simulink model "BenchmarkModel_Dynamic_TestCase"  (R2020a)
settings: Solver=ode45  StartTime=0.0  StopTime=5  RelTol=1e-3
undefined symbols (not defined in the file): Angle, D1, Delta, find_system, Magnitude
libraries: powerlib x91, powerlib_meascontrol x31, simulink x6, dspsrcs4 x3, dspsigops x2, sps_avr x1
(part 2 of 3)

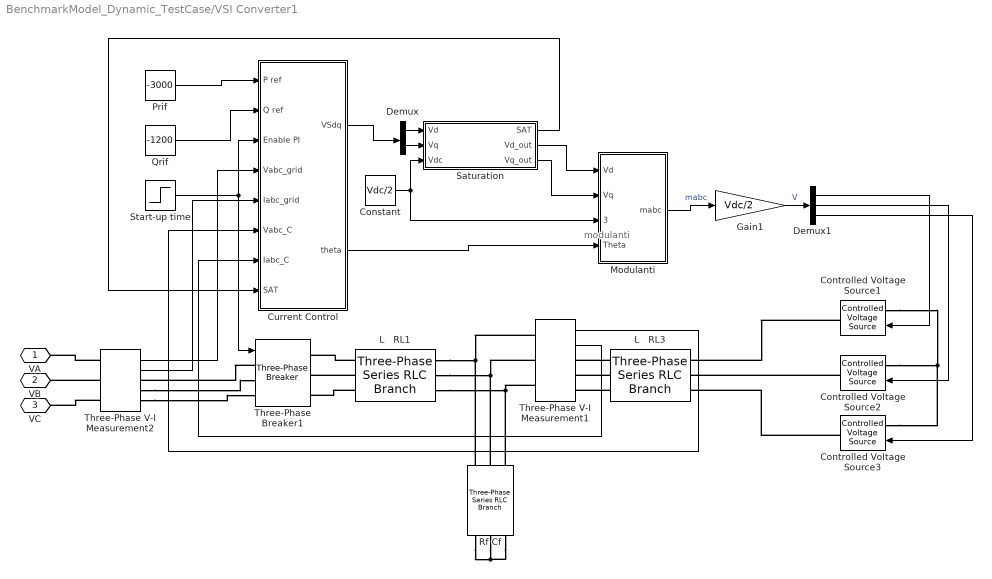
== system BenchmarkModel_Dynamic_TestCase/VSI Converter1 ==
  note: modulanti
  Constant : Constant  Value=Vdc/2
  Controlled Voltage Source1 : powerlib/Electrical Sources/Controlled Voltage Source  Initialize=on  Source_Type=DC  Amplitude=0  Phase=0  Frequency=0  Measurements=None
  Controlled Voltage Source2 : powerlib/Electrical Sources/Controlled Voltage Source  Initialize=on  Source_Type=DC  Amplitude=0  Phase=0  Frequency=0  Measurements=None
  Controlled Voltage Source3 : powerlib/Electrical Sources/Controlled Voltage Source  Initialize=on  Source_Type=DC  Amplitude=0  Phase=0  Frequency=0  Measurements=None
  Current Control : Subsystem
  Demux : Demux  Outputs=2
  Demux1 : Demux  Outputs=3
  Gain1 : Gain  Gain=Vdc/2
  L	  RL1 : powerlib/Elements/Three-Phase Series RLC Branch  LConnTagsString=A|B|C  RConnTagsString=A|B|C  BranchType=L  Resistance=0  Inductance=Lf  Capacitance=100e-6  Measurements=Branch voltages
  L	  RL3 : powerlib/Elements/Three-Phase Series RLC Branch  LConnTagsString=A|B|C  RConnTagsString=A|B|C  BranchType=RL  Resistance=10e-3  Inductance=L1t  Capacitance=100e-6  Measurements=None
  Modulanti : Subsystem
  Prif : Constant  Value=-3000
  Qrif : Constant  Value=-1200
  "Rf Cf  " : powerlib/Elements/Three-Phase Series RLC Branch  LConnTagsString=A|B|C  RConnTagsString=A|B|C  BranchType=RC  Resistance=1e-3  Inductance=1e-3  Capacitance=Cf  Measurements=Branch voltages
  Saturation : MATLAB Function  TreatAsAtomicUnit=on
  Start-up time : Step  Time=0.05  SampleTime=0
  Three-Phase V-I Measurement1 : powerlib/Measurements/Three-Phase V-I Measurement  VoltageMeasurement=phase-to-phase  SetLabelV=off  LabelV=Vabc  Vpu=off  VpuLL=off  CurrentMeasurement=yes  SetLabelI=off  LabelI=Iabc  Ipu=off  Pbase=100e6  Vbase=500e3  OutputType=Complex  PhasorSimulation=off  PSBequivalent=0
  Three-Phase V-I Measurement2 : powerlib/Measurements/Three-Phase V-I Measurement  VoltageMeasurement=phase-to-phase  SetLabelV=off  LabelV=Vabc  Vpu=off  VpuLL=off  CurrentMeasurement=yes  SetLabelI=off  LabelI=Iabc  Ipu=off  Pbase=100e6  Vbase=500e3  OutputType=Complex  PhasorSimulation=off  PSBequivalent=0
  Three-Phase Breaker1 : powerlib/Elements/Three-Phase Breaker  InitialState=open  SwitchA=on  SwitchB=on  SwitchC=on  SwitchTimes="[1/60  5/60]"  External=on  BreakerResistance=0.001  SnubberResistance=1e6  SnubberCapacitance=inf  Measurements=None
  VA : PMIOPort  Side=Left
  VB : PMIOPort  Port=2  Side=Left
  VC : PMIOPort  Port=3  Side=Left
  wires:
  Constant/1 -> Modulanti/3(Vdcbus), Saturation/3(Vdc)
  Saturation/1(SAT) -> Current Control/8(SAT)
  Start-up time/1 -> Three-Phase Breaker1/1, Current Control/3(Enable PI)
  Current Control/1(VSdq) -> Demux/1
  Demux/1 -> Saturation/1(Vd)
  Demux/2 -> Saturation/2(Vq)
  Saturation/2(Vd_out) -> Modulanti/1(Vd)
  Saturation/3(Vq_out) -> Modulanti/2(Vq)
  Modulanti/1(mabc) -> Gain1/1  "mabc"
  Demux1/1 -> Controlled Voltage Source1/1
  Demux1/2 -> Controlled Voltage Source2/1
  Demux1/3 -> Controlled Voltage Source3/1
  Gain1/1 -> Demux1/1  "V"
  Prif/1 -> Current Control/1(P ref)
  Qrif/1 -> Current Control/2(Q ref)
  Three-Phase V-I Measurement2/2 -> Current Control/5(Iabc_grid)
  Three-Phase V-I Measurement2/1 -> Current Control/4(Vabc_grid)
  Three-Phase V-I Measurement1/2 -> Current Control/7(Iabc_C)
  Three-Phase V-I Measurement1/1 -> Current Control/6(Vabc_C)
  Current Control/2(theta) -> Modulanti/4(Theta)
  connections:
  L	  RL1/LConn3 -- Three-Phase V-I Measurement1/LConn3 -- "Rf Cf  "/LConn3
  "Rf Cf  "/RConn1 -- "Rf Cf  "/RConn3 -- "Rf Cf  "/RConn2
  L	  RL1/LConn1 -- Three-Phase V-I Measurement1/LConn1 -- "Rf Cf  "/LConn1
  L	  RL1/LConn2 -- Three-Phase V-I Measurement1/LConn2 -- "Rf Cf  "/LConn2
  Controlled Voltage Source3/RConn1 -- L	  RL3/LConn3
  Controlled Voltage Source1/RConn1 -- L	  RL3/LConn1
  L	  RL1/RConn1 -- Three-Phase Breaker1/RConn1
  L	  RL1/RConn2 -- Three-Phase Breaker1/RConn2
  L	  RL1/RConn3 -- Three-Phase Breaker1/RConn3
  Three-Phase V-I Measurement2/LConn3 -- VC/RConn1
  Three-Phase V-I Measurement2/LConn2 -- VB/RConn1
  Three-Phase V-I Measurement2/LConn1 -- VA/RConn1
  Controlled Voltage Source2/LConn1 -- Controlled Voltage Source1/LConn1 -- Controlled Voltage Source3/LConn1
  Controlled Voltage Source2/RConn1 -- L	  RL3/LConn2
  Three-Phase Breaker1/LConn1 -- Three-Phase V-I Measurement2/RConn1
  L	  RL3/RConn1 -- Three-Phase V-I Measurement1/RConn1
  L	  RL3/RConn2 -- Three-Phase V-I Measurement1/RConn2
  L	  RL3/RConn3 -- Three-Phase V-I Measurement1/RConn3
  Three-Phase V-I Measurement2/RConn2 -- Three-Phase Breaker1/LConn2
  Three-Phase V-I Measurement2/RConn3 -- Three-Phase Breaker1/LConn3

== system BenchmarkModel_Dynamic_TestCase/Zero-crossing detector ==
  Ground2 : powerlib/Elements/Ground  LConnTagsString=a
  To Workspace5 : ToWorkspace  VariableName=Crossing_Inv  SaveFormat=Timeseries  SampleTime=-1
  Voltage Measurement2 : powerlib/Measurements/Voltage Measurement  PhasorSimulation=off  OutputType=Complex  PSBequivalent=0
  Zero Crossing1 : dspsigops/Zero Crossing  InputProcessing=Columns as channels (frame based)
      settings: SourceProductBaseCode=DS
  v : PMIOPort  Side=Left
  wires:
  Voltage Measurement2/1 -> Zero Crossing1/1
  Zero Crossing1/1 -> To Workspace5/1
  connections:
  Ground2/LConn1 -- Voltage Measurement2/LConn2
  v/RConn1 -- Voltage Measurement2/LConn1

== system BenchmarkModel_Dynamic_TestCase/ZeroCrossing Detector ==
  Ground1 : powerlib/Elements/Ground  LConnTagsString=a
  To Workspace4 : ToWorkspace  VariableName=Crossing  SaveFormat=Timeseries  SampleTime=-1
  Voltage Measurement1 : powerlib/Measurements/Voltage Measurement  PhasorSimulation=off  OutputType=Complex  PSBequivalent=0
  Zero Crossing : dspsigops/Zero Crossing  InputProcessing=Columns as channels (frame based)
      settings: SourceProductBaseCode=DS
  fr : PMIOPort  Side=Left
  wires:
  Zero Crossing/1 -> To Workspace4/1
  Voltage Measurement1/1 -> Zero Crossing/1
  connections:
  Ground1/LConn1 -- Voltage Measurement1/LConn2
  fr/RConn1 -- Voltage Measurement1/LConn1

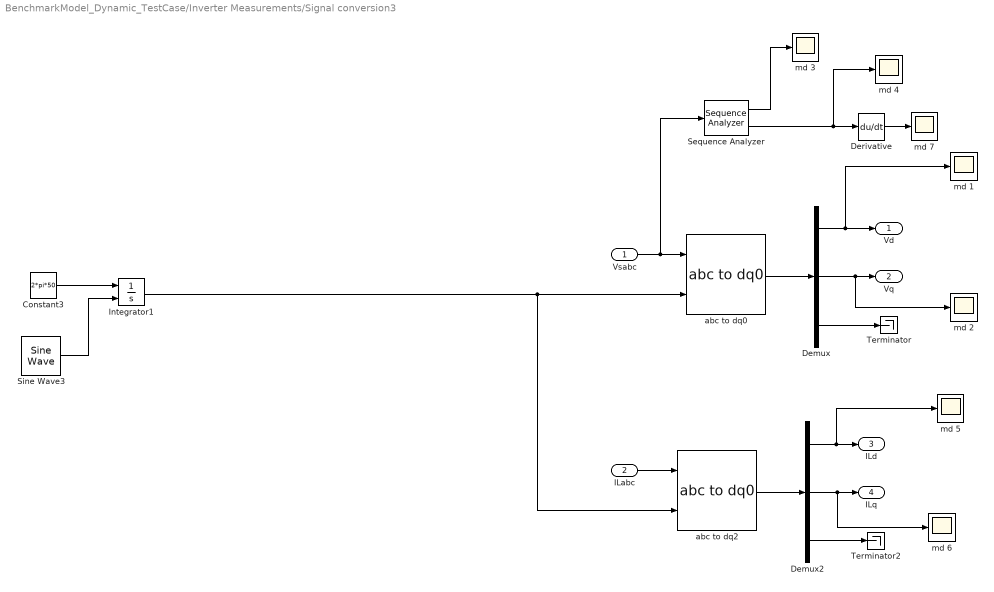
== system BenchmarkModel_Dynamic_TestCase/Inverter Measurements/Signal conversion3 ==
  Vsabc : Inport
  ILabc : Inport  Port=2
  Constant3 : Constant  Value=2*pi*50
  Demux : Demux  Outputs=3
  Demux2 : Demux  Outputs=3
  Derivative : Derivative
  Integrator1 : Integrator  ExternalReset=rising
  Sequence Analyzer : powerlib_meascontrol/Measurements/Sequence Analyzer  Freq=50  n=1  seq=Positive Negative Zero  InInit=[1, 0]  Ts=0
      settings: SourceProductBaseCode=PS
  Sine Wave3 : dspsrcs4/Sine Wave  Amplitude=1  Frequency=50  Phase=0  SampleMode=Continuous  OutComplex=Real  CompMethod=Trigonometric fcn  TableSize=Speed  SampleTime=5e-6  SamplesPerFrame=1  ResetState=Restart at time zero  OutputFrames=on  dataType=double  wordLen=16  udDataType=sfix(16)  fracBitsMode=Best precision  numFracBits=15  OutDataTypeStr=double  LastOutDataTypeStr=double
  Terminator : Terminator
  Terminator2 : Terminator
  abc to dq0 : powerlib_meascontrol/Transformations/abc to dq0  Alignment=90 degrees behind phase A axis
  abc to dq2 : powerlib_meascontrol/Transformations/abc to dq0  Alignment=90 degrees behind phase A axis
  md {1..7} (7 alike) : Scope
  Vd : Outport
  Vq : Outport  Port=2
  ILd : Outport  Port=3
  ILq : Outport  Port=4
  wires:
  Vsabc/1 -> Sequence Analyzer/1, abc to dq0/1
  Demux2/1 -> ILd/1, md 5/1
  Integrator1/1 -> abc to dq2/2, abc to dq0/2
  ILabc/1 -> abc to dq2/1
  Demux2/3 -> Terminator2/1
  Demux/3 -> Terminator/1
  Constant3/1 -> Integrator1/1
  abc to dq0/1 -> Demux/1
  abc to dq2/1 -> Demux2/1
  Demux/1 -> Vd/1, md 1/1
  Demux/2 -> Vq/1, md 2/1
  Demux2/2 -> ILq/1, md 6/1
  Sine Wave3/1 -> Integrator1/2
  Sequence Analyzer/1 -> md 3/1
  Sequence Analyzer/2 -> Derivative/1, md 4/1
  Derivative/1 -> md 7/1

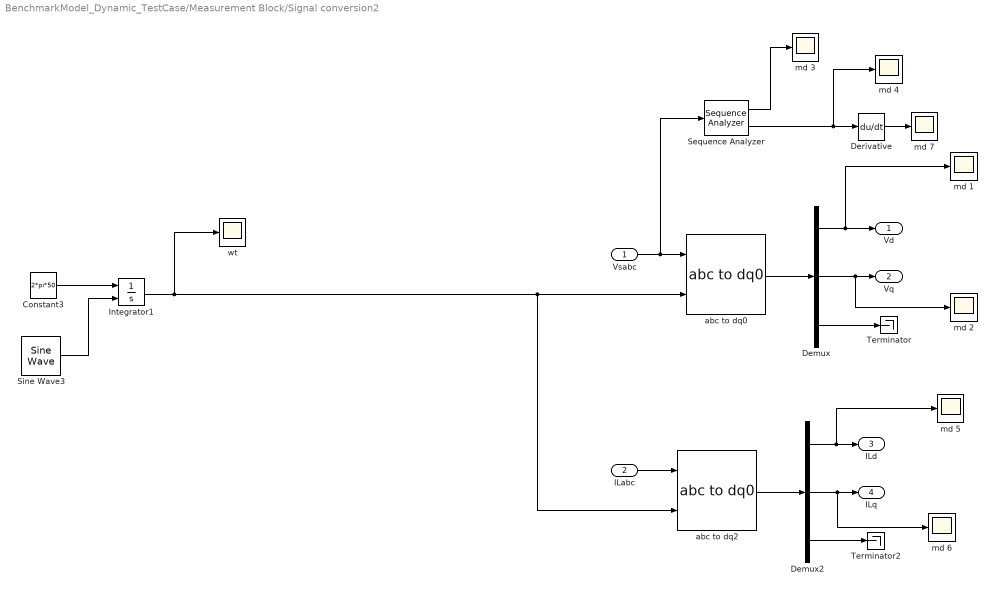
== system BenchmarkModel_Dynamic_TestCase/Measurement Block/Signal conversion2 ==
  Vsabc : Inport
  ILabc : Inport  Port=2
  Constant3 : Constant  Value=2*pi*50
  Demux : Demux  Outputs=3
  Demux2 : Demux  Outputs=3
  Derivative : Derivative
  Integrator1 : Integrator  ExternalReset=rising
  Sequence Analyzer : powerlib_meascontrol/Measurements/Sequence Analyzer  Freq=50  n=1  seq=Positive Negative Zero  InInit=[1, 0]  Ts=0
      settings: SourceProductBaseCode=PS
  Sine Wave3 : dspsrcs4/Sine Wave  Amplitude=1  Frequency=50  Phase=0  SampleMode=Continuous  OutComplex=Real  CompMethod=Trigonometric fcn  TableSize=Speed  SampleTime=5e-6  SamplesPerFrame=1  ResetState=Restart at time zero  OutputFrames=on  dataType=double  wordLen=16  udDataType=sfix(16)  fracBitsMode=Best precision  numFracBits=15  OutDataTypeStr=double  LastOutDataTypeStr=double
  Terminator : Terminator
  Terminator2 : Terminator
  abc to dq0 : powerlib_meascontrol/Transformations/abc to dq0  Alignment=90 degrees behind phase A axis
  abc to dq2 : powerlib_meascontrol/Transformations/abc to dq0  Alignment=90 degrees behind phase A axis
  md {1..7} (7 alike) : Scope
  wt : Scope
  Vd : Outport
  Vq : Outport  Port=2
  ILd : Outport  Port=3
  ILq : Outport  Port=4
  wires:
  Vsabc/1 -> Sequence Analyzer/1, abc to dq0/1
  Demux2/1 -> ILd/1, md 5/1
  Integrator1/1 -> abc to dq2/2, abc to dq0/2, wt/1
  ILabc/1 -> abc to dq2/1
  Demux2/3 -> Terminator2/1
  Demux/3 -> Terminator/1
  Constant3/1 -> Integrator1/1
  abc to dq0/1 -> Demux/1
  abc to dq2/1 -> Demux2/1
  Demux/1 -> Vd/1, md 1/1
  Demux/2 -> Vq/1, md 2/1
  Demux2/2 -> ILq/1, md 6/1
  Sine Wave3/1 -> Integrator1/2
  Sequence Analyzer/1 -> md 3/1
  Sequence Analyzer/2 -> Derivative/1, md 4/1
  Derivative/1 -> md 7/1

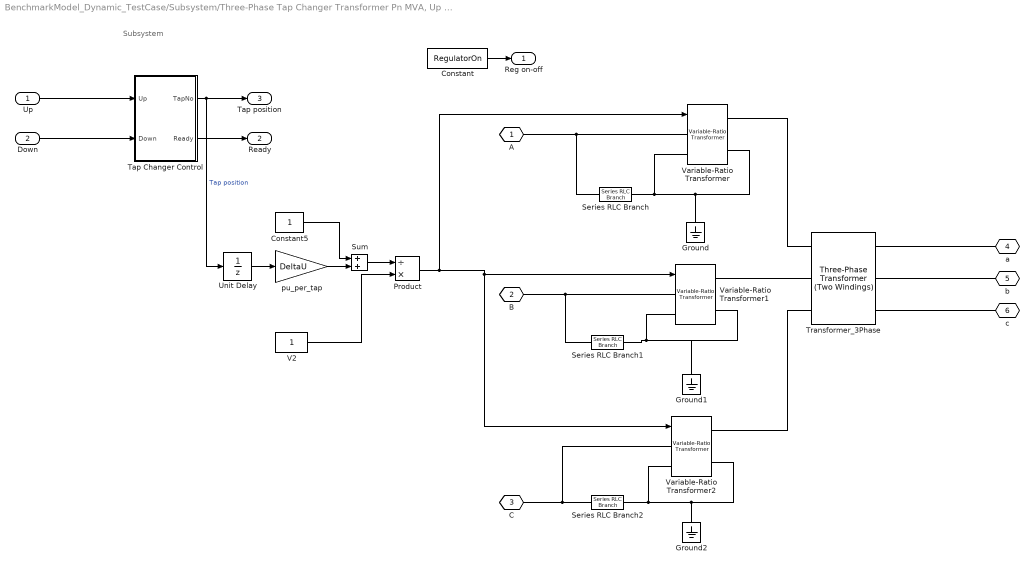
== system BenchmarkModel_Dynamic_TestCase/Subsystem/Three-Phase Tap Changer Transformer Pn MVA, Up // Us kV ==
  note: Subsystem
  Up : Inport
  Down : Inport  Port=2
  Constant : Constant  Value=RegulatorOn
  Constant5 : Constant
  Ground : powerlib/Elements/Ground  LConnTagsString=a
  Ground1 : powerlib/Elements/Ground  LConnTagsString=a
  Ground2 : powerlib/Elements/Ground  LConnTagsString=a
  Product : Product  Inputs=/*
  Series RLC Branch : powerlib/Elements/Series RLC Branch  LConnTagsString=__new0  RConnTagsString=__new0  BranchType=R  Resistance=1e7  Inductance=1e-3  SetiL0=off  InitialCurrent=0  Capacitance=1e-6  Setx0=off  InitialVoltage=0  Measurements=None
  Series RLC Branch1 : powerlib/Elements/Series RLC Branch  LConnTagsString=__new0  RConnTagsString=__new0  BranchType=R  Resistance=1e7  Inductance=1e-3  SetiL0=off  InitialCurrent=0  Capacitance=1e-6  Setx0=off  InitialVoltage=0  Measurements=None
  Series RLC Branch2 : powerlib/Elements/Series RLC Branch  LConnTagsString=__new0  RConnTagsString=__new0  BranchType=R  Resistance=1e7  Inductance=1e-3  SetiL0=off  InitialCurrent=0  Capacitance=1e-6  Setx0=off  InitialVoltage=0  Measurements=None
  Sum : Sum
  Tap Changer Control : Subsystem  mask(Tap Changer Control){MinMaxTap=TapMinMax, InitialPosition=InitialTap, MecDelay=TapSelectionTime}
      mask prompts: MinMaxTap "Minimum and maximum tap number [ Min  Max ] :"; InitialPosition "Initial tap position"; MecDelay "Mechanical delay time"
      mask init:
      | if MecDelay<=0,
      | 	MecDelay=1/60;
      | end
  Transformer_3Phase : powerlib/Elements/Three-Phase Transformer (Two Windings)  Winding1Connection=Yg  Winding2Connection=Delta (D1)  CoreType=Three single-phase transformers  SetSaturation=off  Hysteresis=off  DataFile='hysteresis'  SetInitialFlux=off  Measurements=Fluxes and magnetization currents ( Imag )  UNITS=pu  NominalPower=NominalParameters  Winding1=Winding1  Winding2=Winding2  Rm=Rmpu  Lm=Lmpu  L0=0.5  Saturation=[ 0,0 ; 0.0024,1.2 ; 1.0,1.52 ]  InitialFluxes=[ 0.8 , -0.8 , 0.7 ]  BreakLoop=off  DiscreteSolver=Trapezoidal iterative  DataType=off  TransfoNumber=1
  Unit Delay : UnitDelay  InitialCondition=InitialTap  SampleTime=50e-6  HasFrameUpgradeWarning=on
  V2 : Constant
  Variable-Ratio Transformer : powerlib/Elements/Variable-Ratio Transformer
      settings: SourceProductBaseCode=PS
  Variable-Ratio Transformer1 : powerlib/Elements/Variable-Ratio Transformer
      settings: SourceProductBaseCode=PS
  Variable-Ratio Transformer2 : powerlib/Elements/Variable-Ratio Transformer
      settings: SourceProductBaseCode=PS
  pu_per_tap : Gain  Gain=DeltaU
  A : PMIOPort  Tag=PMCPort  Side=Left
  B : PMIOPort  Tag=PMCPort  Port=2  Side=Left
  C : PMIOPort  Tag=PMCPort  Port=3  Side=Left
  a : PMIOPort  Tag=PMCPort  Port=4  Side=Right
  b : PMIOPort  Tag=PMCPort  Port=5  Side=Right
  c : PMIOPort  Tag=PMCPort  Port=6  Side=Right
  Reg on-off : Outport
  Ready : Outport  Port=2
  Tap position : Outport  Port=3
  wires:
  Constant/1 -> Reg on-off/1
  Tap Changer Control/2(Ready) -> Ready/1
  Constant5/1 -> Sum/1
  Up/1 -> Tap Changer Control/1("Up ")
  Tap Changer Control/1(TapNo) -> Unit Delay/1, Tap position/1  "Tap position"
  Unit Delay/1 -> pu_per_tap/1
  Down/1 -> Tap Changer Control/2("Down ")
  Sum/1 -> Product/1
  V2/1 -> Product/2
  pu_per_tap/1 -> Sum/2
  Product/1 -> Variable-Ratio Transformer2/1, Variable-Ratio Transformer1/1, Variable-Ratio Transformer/1
  connections:
  Transformer_3Phase/RConn1 -- a/RConn1
  Transformer_3Phase/RConn2 -- b/RConn1
  Transformer_3Phase/RConn3 -- c/RConn1
  Transformer_3Phase/LConn2 -- Variable-Ratio Transformer1/RConn1
  Transformer_3Phase/LConn3 -- Variable-Ratio Transformer2/RConn1
  Transformer_3Phase/LConn1 -- Variable-Ratio Transformer/RConn1
  Series RLC Branch1/LConn1 -- B/RConn1 -- Variable-Ratio Transformer1/LConn1
  Variable-Ratio Transformer/LConn1 -- A/RConn1 -- Series RLC Branch/LConn1
  Series RLC Branch2/LConn1 -- Variable-Ratio Transformer2/LConn1 -- C/RConn1
  Ground2/LConn1 -- Variable-Ratio Transformer2/LConn2 -- Series RLC Branch2/RConn1 -- Variable-Ratio Transformer2/RConn2
  Series RLC Branch1/RConn1 -- Variable-Ratio Transformer1/RConn2 -- Ground1/LConn1 -- Variable-Ratio Transformer1/LConn2
  Ground/LConn1 -- Variable-Ratio Transformer/LConn2 -- Series RLC Branch/RConn1 -- Variable-Ratio Transformer/RConn2

== system BenchmarkModel_Dynamic_TestCase/Subsystem/Voltage regulator ==
  Vmes (pu) : Inport
  Ready : Inport  Port=2
  RegOn : Inport  Port=3
  Dead Zone : DeadZone  LowerValue=-DeadBand/2  UpperValue=+DeadBand/2  SaturateOnIntegerOverflow=on
  Discrete Variable Time Delay1 : powerlib_meascontrol/Additional Components/Discrete Variable Time Delay  MaxDelay=3/60+50e-6  InitialValue=1  Ts=50e-6  DFT=on
      settings: SourceProductBaseCode=PS
  Logical Operator : Logic  AllPortsSameDT=off
  Logical Operator1 : Logic  AllPortsSameDT=off
  On Delay : powerlib_meascontrol/Logic/On Delay  DelayType=On delay  delay=TimeDelay  ic=0  Ts=50e-6
  On Delay1 : powerlib_meascontrol/Logic/On Delay  DelayType=On delay  delay=TimeDelay  ic=0  Ts=50e-6
  Relational Operator : RelationalOperator  Operator=<  RndMeth=Nearest
  Relational Operator1 : RelationalOperator  Operator=>  RndMeth=Nearest
  Scope : Scope  Commented=on  NumInputPorts=2
  Sum : Sum  Inputs=|+-  SaturateOnIntegerOverflow=on
  Switch : Switch  Threshold=1.5  SaturateOnIntegerOverflow=on
  Vref : Constant  Value=Vref
  Vref1 : Constant  Value=0
  Vref2 : Constant  Value=0
  Vref3 : Constant  Value=0
  Vref4 : Constant  Value=3/60
  Up : Outport  VectorParamsAs1DForOutWhenUnconnected=off
  Down : Outport  Port=2  VectorParamsAs1DForOutWhenUnconnected=off
  wires:
  Vref4/1 -> Discrete Variable Time Delay1/2
  Discrete Variable Time Delay1/1 -> Logical Operator/2, Logical Operator1/1
  Vref3/1 -> Relational Operator1/2
  On Delay1/1 -> Down/1
  Logical Operator1/1 -> On Delay1/1
  Relational Operator1/1 -> Logical Operator1/2
  On Delay/1 -> Up/1
  Logical Operator/1 -> On Delay/1
  Ready/1 -> Discrete Variable Time Delay1/1
  Relational Operator/1 -> Logical Operator/1
  Vref1/1 -> Relational Operator/2
  Dead Zone/1 -> Scope/2, Relational Operator/1, Relational Operator1/1
  Vmes (pu)/1 -> Sum/2
  Vref/1 -> Sum/1
  Sum/1 -> Switch/1
  Switch/1 -> Scope/1, Dead Zone/1  "bfor"
  RegOn/1 -> Switch/2
  Vref2/1 -> Switch/3

== system BenchmarkModel_Dynamic_TestCase/Subsystem1/POWER CONVERTER1 ==
  phase3 : Inport
  Add : Sum
  Add2 : Sum
  Add4 : Sum
  Ampl : Constant  Value=20000*sqrt(2)/sqrt(3)
  Product : Product
  Product1 : Product
  Product2 : Product
  Sin : Trigonometry
  Sin1 : Trigonometry
  Sin2 : Trigonometry
  phase : Constant  Value=0
  phase1 : Constant  Value=-120*pi/180
  phase2 : Constant  Value=-240*pi/180
  Phase A : Outport
  Phase B : Outport  Port=2
  Phase C : Outport  Port=3
  wires:
  phase/1 -> Add/1
  Add/1 -> Sin/1
  phase1/1 -> Add2/1
  Add2/1 -> Sin1/1
  phase2/1 -> Add4/1
  Add4/1 -> Sin2/1
  phase3/1 -> Add/2, Add4/2, Add2/2
  Ampl/1 -> Product2/1, Product1/1, Product/1
  Product1/1 -> Phase B/1
  Product2/1 -> Phase C/1
  Product/1 -> Phase A/1
  Sin/1 -> Product/2
  Sin1/1 -> Product1/2
  Sin2/1 -> Product2/2

== system BenchmarkModel_Dynamic_TestCase/Subsystem1/Phase calculator1 ==
  f1 : Inport
  Add3 : Sum  Inputs=+-
  Gain : Gain  Gain=2*pi
  Integrator : Integrator
  f : Constant  Value=0
  phase : Outport
  wires:
  Add3/1 -> Gain/1
  f/1 -> Add3/2
  f1/1 -> Add3/1
  Integrator/1 -> phase/1
  Gain/1 -> Integrator/1

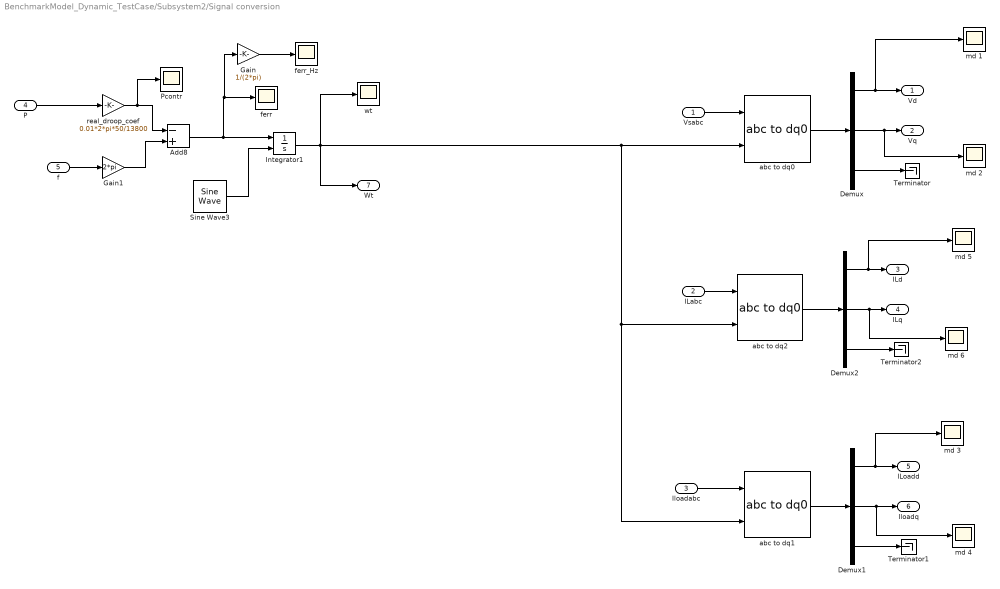
== system BenchmarkModel_Dynamic_TestCase/Subsystem2/Signal conversion ==
  Vsabc : Inport
  ILabc : Inport  Port=2
  Iloadabc : Inport  Port=3
  P : Inport  Port=4
  f : Inport  Port=5
  Add8 : Sum  Inputs=-+
  Demux : Demux  Outputs=3
  Demux1 : Demux  Outputs=3
  Demux2 : Demux  Outputs=3
  Gain : Gain  Gain=1/(2*pi)
  Gain1 : Gain  Gain=2*pi
  Integrator1 : Integrator  ExternalReset=rising
  Pcontr : Scope
  Sine Wave3 : dspsrcs4/Sine Wave  Amplitude=1  Frequency=50  Phase=0  SampleMode=Continuous  OutComplex=Real  CompMethod=Trigonometric fcn  TableSize=Speed  SampleTime=5e-6  SamplesPerFrame=1  ResetState=Restart at time zero  OutputFrames=on  dataType=double  wordLen=16  udDataType=sfix(16)  fracBitsMode=Best precision  numFracBits=15  OutDataTypeStr=double  LastOutDataTypeStr=double
  Terminator : Terminator
  Terminator1 : Terminator
  Terminator2 : Terminator
  abc to dq0 : powerlib_meascontrol/Transformations/abc to dq0  Alignment=90 degrees behind phase A axis
  abc to dq1 : powerlib_meascontrol/Transformations/abc to dq0  Alignment=90 degrees behind phase A axis
  abc to dq2 : powerlib_meascontrol/Transformations/abc to dq0  Alignment=90 degrees behind phase A axis
  ferr : Scope
  ferr_Hz : Scope
  md {1..6} (6 alike) : Scope
  real_droop_coef : Gain  Gain=0.01*2*pi*50/13800
  wt : Scope
  Vd : Outport
  Vq : Outport  Port=2
  ILd : Outport  Port=3
  ILq : Outport  Port=4
  ILoadd : Outport  Port=5
  Iloadq : Outport  Port=6
  Wt : Outport  Port=7
  wires:
  Vsabc/1 -> abc to dq0/1
  Demux2/1 -> ILd/1, md 5/1
  Integrator1/1 -> Wt/1, abc to dq1/2, abc to dq2/2, abc to dq0/2, wt/1
  Demux1/3 -> Terminator1/1
  Demux1/1 -> ILoadd/1, md 3/1
  Iloadabc/1 -> abc to dq1/1
  ILabc/1 -> abc to dq2/1
  Demux1/2 -> Iloadq/1, md 4/1
  Demux2/3 -> Terminator2/1
  Demux/3 -> Terminator/1
  abc to dq1/1 -> Demux1/1
  abc to dq0/1 -> Demux/1
  abc to dq2/1 -> Demux2/1
  Demux/1 -> Vd/1, md 1/1
  Demux/2 -> Vq/1, md 2/1
  Demux2/2 -> ILq/1, md 6/1
  Sine Wave3/1 -> Integrator1/2
  P/1 -> real_droop_coef/1
  Gain1/1 -> Add8/2
  real_droop_coef/1 -> Pcontr/1, Add8/1
  Add8/1 -> Gain/1, ferr/1, Integrator1/1
  Gain/1 -> ferr_Hz/1
  f/1 -> Gain1/1

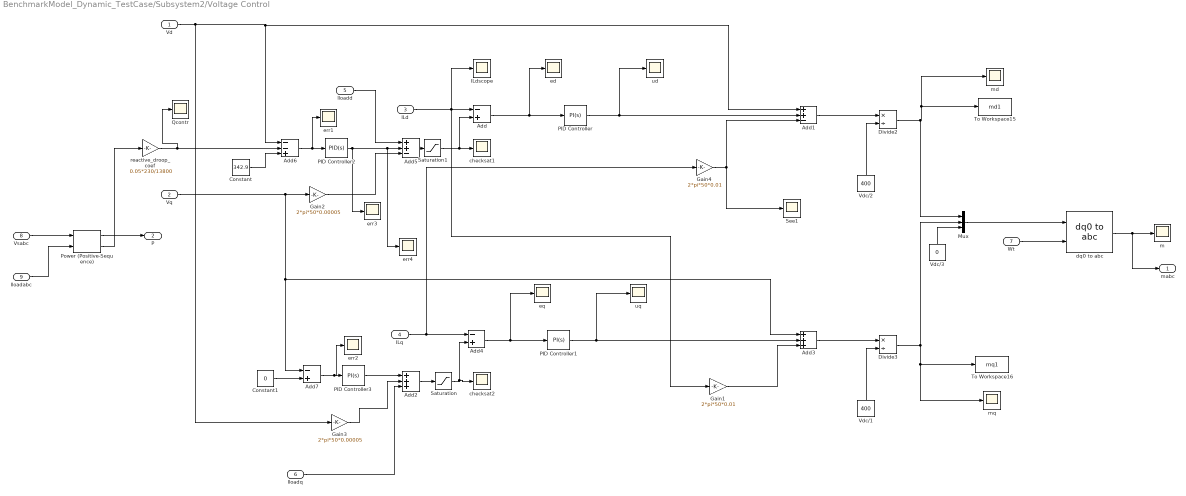
== system BenchmarkModel_Dynamic_TestCase/Subsystem2/Voltage Control ==
  Vd : Inport
  Vq : Inport  Port=2
  ILd : Inport  Port=3
  ILq : Inport  Port=4
  Iloadd : Inport  Port=5
  Iloadq : Inport  Port=6
  Wt : Inport  Port=7
  Vsabc : Inport  Port=8
  Iloadabc : Inport  Port=9
  Add : Sum  Inputs=-+
  Add1 : Sum  Inputs=++-
  Add2 : Sum  Inputs=+++
  Add3 : Sum  Inputs=+++
  Add4 : Sum  Inputs=-+
  Add5 : Sum  Inputs=++-
  Add6 : Sum  Inputs=--+
  Add7 : Sum  Inputs=-+
  Constant : Constant  Value=342.9
  Constant1 : Constant  Value=0
  Divide2 : Product  Inputs=*/
  Divide3 : Product  Inputs=*/
  Gain1 : Gain  Gain=2*pi*50*0.01
  Gain2 : Gain  Gain=2*pi*50*0.00005
  Gain3 : Gain  Gain=2*pi*50*0.00005
  Gain4 : Gain  Gain=2*pi*50*0.01
  ILdscope : Scope
  Mux : Mux  Inputs=3
  PID Controller : simulink/Continuous/PID Controller  Controller=PI  Form=Parallel  TimeDomain=Continuous-time  UseExternalTs=off  SampleTime=-1  IntegratorMethod=Forward Euler  FilterMethod=Forward Euler  ControllerParametersSource=internal  P=20  I=100  D=0  UseFilter=on  N=100  TunerSelectOption=Transfer Function Based (PID Tuner App)  InitialConditionSource=internal  InitialConditionForIntegrator=0  InitialConditionForFilter=0  DifferentiatorICPrevScaledInput=0  ExternalReset=none  TrackingMode=off  Kt=1  LimitOutput=off  UpperSaturationLimit=inf  LowerSaturationLimit=-inf  LinearizeAsGain=on  AntiWindupMode=none  Kb=1  POutMin=[]  POutMax=[]  IOutMin=[]  IOutMax=[]  DOutMin=[]  DOutMax=[]  NOutMin=[]  NOutMax=[]  SumOutMin=[]  SumOutMax=[]  SaturationOutMin=[]  SaturationOutMax=[]  PParamMin=[]  PParamMax=[]  IParamMin=[]  IParamMax=[]  DParamMin=[]  DParamMax=[]  NParamMin=[]  NParamMax=[]  KbParamMin=[]  KbParamMax=[]  KtParamMin=[]  KtParamMax=[]  KbOutMin=[]  KbOutMax=[]  KtOutMin=[]  KtOutMax=[]  IntegratorOutMin=[]  IntegratorOutMax=[]  FilterOutMin=[]  FilterOutMax=[]  SumI1OutMin=[]  SumI1OutMax=[]  SumI2OutMin=[]  SumI2OutMax=[]  SumI3OutMin=[]  SumI3OutMax=[]  SumI4OutMin=[]  SumI4OutMax=[]  SumDOutMin=[]  SumDOutMax=[]  DifferentiatorOutMin=[]  DifferentiatorOutMax=[]  FilterDiffOutCoefMin=[]  FilterDiffOutCoefMax=[]  ReciprocalOutMin=[]  ReciprocalOutMax=[]  SumDenOutMin=[]  SumDenOutMax=[]  SumNumOutMin=[]  SumNumOutMax=[]  DivideOutMin=[]  DivideOutMax=[]  UdiffTsProdOutMin=[]  UdiffTsProdOutMax=[]  NTsProdOutMin=[]  NTsProdOutMax=[]  UintegralTsProdOutMin=[]  UintegralTsProdOutMax=[]  UngainTsProdOutMin=[]  UngainTsProdOutMax=[]  IntegratorContinuousStateAttributes=''  IntegratorStateMustResolveToSignalObject=off  IntegratorRTWStateStorageClass=Auto  FilterContinuousStateAttributes=''  FilterStateMustResolveToSignalObject=off  FilterRTWStateStorageClass=Auto  ParallelPVariant=InternalParameters  IdealPVariant=Disabled  IVariant=InternalParameters  DVariant=Disabled  IntegratorVariant=Continuous  SatVariant=Disabled  AWVariant=Passthrough  PCopyVariant=Disabled  TRVariant=Disabled  FdbkBlocksVariant=Forward  IdealPFdbkVariant=Disabled  SatFdbkVariant=Disabled  DerivativeFilterVariant=Disabled  NVariant=Disabled  NCopyVariant=Disabled_SignalSpec  FilterICVariant=Disabled  IntegratorICVariant=InternalICs  ExternalResetVariant=Disabled  TRSumVariant=Passthrough  SumFdbkVariant=Disabled  SumVariant=Sum_PI  TsampFilterVariant=InternalTs  TsampNgainVariant=Passthrough  TsampIntegralVariant=Passthrough
  PID Controller1 : simulink/Continuous/PID Controller  Controller=PI  Form=Parallel  TimeDomain=Continuous-time  UseExternalTs=off  SampleTime=-1  IntegratorMethod=Forward Euler  FilterMethod=Forward Euler  ControllerParametersSource=internal  P=20  I=100  D=0  UseFilter=on  N=100  TunerSelectOption=Transfer Function Based (PID Tuner App)  InitialConditionSource=internal  InitialConditionForIntegrator=0  InitialConditionForFilter=0  DifferentiatorICPrevScaledInput=0  ExternalReset=none  TrackingMode=off  Kt=1  LimitOutput=off  UpperSaturationLimit=inf  LowerSaturationLimit=-inf  LinearizeAsGain=on  AntiWindupMode=none  Kb=1  POutMin=[]  POutMax=[]  IOutMin=[]  IOutMax=[]  DOutMin=[]  DOutMax=[]  NOutMin=[]  NOutMax=[]  SumOutMin=[]  SumOutMax=[]  SaturationOutMin=[]  SaturationOutMax=[]  PParamMin=[]  PParamMax=[]  IParamMin=[]  IParamMax=[]  DParamMin=[]  DParamMax=[]  NParamMin=[]  NParamMax=[]  KbParamMin=[]  KbParamMax=[]  KtParamMin=[]  KtParamMax=[]  KbOutMin=[]  KbOutMax=[]  KtOutMin=[]  KtOutMax=[]  IntegratorOutMin=[]  IntegratorOutMax=[]  FilterOutMin=[]  FilterOutMax=[]  SumI1OutMin=[]  SumI1OutMax=[]  SumI2OutMin=[]  SumI2OutMax=[]  SumI3OutMin=[]  SumI3OutMax=[]  SumI4OutMin=[]  SumI4OutMax=[]  SumDOutMin=[]  SumDOutMax=[]  DifferentiatorOutMin=[]  DifferentiatorOutMax=[]  FilterDiffOutCoefMin=[]  FilterDiffOutCoefMax=[]  ReciprocalOutMin=[]  ReciprocalOutMax=[]  SumDenOutMin=[]  SumDenOutMax=[]  SumNumOutMin=[]  SumNumOutMax=[]  DivideOutMin=[]  DivideOutMax=[]  UdiffTsProdOutMin=[]  UdiffTsProdOutMax=[]  NTsProdOutMin=[]  NTsProdOutMax=[]  UintegralTsProdOutMin=[]  UintegralTsProdOutMax=[]  UngainTsProdOutMin=[]  UngainTsProdOutMax=[]  IntegratorContinuousStateAttributes=''  IntegratorStateMustResolveToSignalObject=off  IntegratorRTWStateStorageClass=Auto  FilterContinuousStateAttributes=''  FilterStateMustResolveToSignalObject=off  FilterRTWStateStorageClass=Auto  ParallelPVariant=InternalParameters  IdealPVariant=Disabled  IVariant=InternalParameters  DVariant=Disabled  IntegratorVariant=Continuous  SatVariant=Disabled  AWVariant=Passthrough  PCopyVariant=Disabled  TRVariant=Disabled  FdbkBlocksVariant=Forward  IdealPFdbkVariant=Disabled  SatFdbkVariant=Disabled  DerivativeFilterVariant=Disabled  NVariant=Disabled  NCopyVariant=Disabled_SignalSpec  FilterICVariant=Disabled  IntegratorICVariant=InternalICs  ExternalResetVariant=Disabled  TRSumVariant=Passthrough  SumFdbkVariant=Disabled  SumVariant=Sum_PI  TsampFilterVariant=InternalTs  TsampNgainVariant=Passthrough  TsampIntegralVariant=Passthrough
  PID Controller2 : simulink/Continuous/PID Controller  Controller=PID  Form=Ideal  TimeDomain=Continuous-time  UseExternalTs=off  SampleTime=-1  IntegratorMethod=Forward Euler  FilterMethod=Forward Euler  ControllerParametersSource=internal  P=0.6  I=1.5  D=0  UseFilter=on  N=100  TunerSelectOption=Transfer Function Based (PID Tuner App)  InitialConditionSource=internal  InitialConditionForIntegrator=0  InitialConditionForFilter=0  DifferentiatorICPrevScaledInput=0  ExternalReset=none  TrackingMode=off  Kt=1  LimitOutput=off  UpperSaturationLimit=inf  LowerSaturationLimit=-inf  LinearizeAsGain=on  AntiWindupMode=none  Kb=1  POutMin=[]  POutMax=[]  IOutMin=[]  IOutMax=[]  DOutMin=[]  DOutMax=[]  NOutMin=[]  NOutMax=[]  SumOutMin=[]  SumOutMax=[]  SaturationOutMin=[]  SaturationOutMax=[]  PParamMin=[]  PParamMax=[]  IParamMin=[]  IParamMax=[]  DParamMin=[]  DParamMax=[]  NParamMin=[]  NParamMax=[]  KbParamMin=[]  KbParamMax=[]  KtParamMin=[]  KtParamMax=[]  KbOutMin=[]  KbOutMax=[]  KtOutMin=[]  KtOutMax=[]  IntegratorOutMin=[]  IntegratorOutMax=[]  FilterOutMin=[]  FilterOutMax=[]  SumI1OutMin=[]  SumI1OutMax=[]  SumI2OutMin=[]  SumI2OutMax=[]  SumI3OutMin=[]  SumI3OutMax=[]  SumI4OutMin=[]  SumI4OutMax=[]  SumDOutMin=[]  SumDOutMax=[]  DifferentiatorOutMin=[]  DifferentiatorOutMax=[]  FilterDiffOutCoefMin=[]  FilterDiffOutCoefMax=[]  ReciprocalOutMin=[]  ReciprocalOutMax=[]  SumDenOutMin=[]  SumDenOutMax=[]  SumNumOutMin=[]  SumNumOutMax=[]  DivideOutMin=[]  DivideOutMax=[]  UdiffTsProdOutMin=[]  UdiffTsProdOutMax=[]  NTsProdOutMin=[]  NTsProdOutMax=[]  UintegralTsProdOutMin=[]  UintegralTsProdOutMax=[]  UngainTsProdOutMin=[]  UngainTsProdOutMax=[]  IntegratorContinuousStateAttributes=''  IntegratorStateMustResolveToSignalObject=off  IntegratorRTWStateStorageClass=Auto  FilterContinuousStateAttributes=''  FilterStateMustResolveToSignalObject=off  FilterRTWStateStorageClass=Auto  ParallelPVariant=Passthrough  IdealPVariant=InternalParameters  IVariant=InternalParameters  DVariant=InternalParameters  IntegratorVariant=Continuous  SatVariant=Disabled  AWVariant=Passthrough  PCopyVariant=Disabled  TRVariant=Disabled  FdbkBlocksVariant=Forward  IdealPFdbkVariant=Disabled  SatFdbkVariant=Disabled  DerivativeFilterVariant=ContFilter  NVariant=InternalParameters  NCopyVariant=Disabled  FilterICVariant=InternalICsFilter  IntegratorICVariant=InternalICs  ExternalResetVariant=Disabled  TRSumVariant=Passthrough  SumFdbkVariant=Disabled  SumVariant=Sum_PID  TsampFilterVariant=InternalTs  TsampNgainVariant=Passthrough  TsampIntegralVariant=Passthrough
  PID Controller3 : simulink/Continuous/PID Controller  Controller=PI  Form=Ideal  TimeDomain=Continuous-time  UseExternalTs=off  SampleTime=-1  IntegratorMethod=Forward Euler  FilterMethod=Forward Euler  ControllerParametersSource=internal  P=0.5  I=10  D=0  UseFilter=on  N=100  TunerSelectOption=Transfer Function Based (PID Tuner App)  InitialConditionSource=internal  InitialConditionForIntegrator=0  InitialConditionForFilter=0  DifferentiatorICPrevScaledInput=0  ExternalReset=none  TrackingMode=off  Kt=1  LimitOutput=off  UpperSaturationLimit=inf  LowerSaturationLimit=-inf  LinearizeAsGain=on  AntiWindupMode=none  Kb=1  POutMin=[]  POutMax=[]  IOutMin=[]  IOutMax=[]  DOutMin=[]  DOutMax=[]  NOutMin=[]  NOutMax=[]  SumOutMin=[]  SumOutMax=[]  SaturationOutMin=[]  SaturationOutMax=[]  PParamMin=[]  PParamMax=[]  IParamMin=[]  IParamMax=[]  DParamMin=[]  DParamMax=[]  NParamMin=[]  NParamMax=[]  KbParamMin=[]  KbParamMax=[]  KtParamMin=[]  KtParamMax=[]  KbOutMin=[]  KbOutMax=[]  KtOutMin=[]  KtOutMax=[]  IntegratorOutMin=[]  IntegratorOutMax=[]  FilterOutMin=[]  FilterOutMax=[]  SumI1OutMin=[]  SumI1OutMax=[]  SumI2OutMin=[]  SumI2OutMax=[]  SumI3OutMin=[]  SumI3OutMax=[]  SumI4OutMin=[]  SumI4OutMax=[]  SumDOutMin=[]  SumDOutMax=[]  DifferentiatorOutMin=[]  DifferentiatorOutMax=[]  FilterDiffOutCoefMin=[]  FilterDiffOutCoefMax=[]  ReciprocalOutMin=[]  ReciprocalOutMax=[]  SumDenOutMin=[]  SumDenOutMax=[]  SumNumOutMin=[]  SumNumOutMax=[]  DivideOutMin=[]  DivideOutMax=[]  UdiffTsProdOutMin=[]  UdiffTsProdOutMax=[]  NTsProdOutMin=[]  NTsProdOutMax=[]  UintegralTsProdOutMin=[]  UintegralTsProdOutMax=[]  UngainTsProdOutMin=[]  UngainTsProdOutMax=[]  IntegratorContinuousStateAttributes=''  IntegratorStateMustResolveToSignalObject=off  IntegratorRTWStateStorageClass=Auto  FilterContinuousStateAttributes=''  FilterStateMustResolveToSignalObject=off  FilterRTWStateStorageClass=Auto  ParallelPVariant=Passthrough  IdealPVariant=InternalParameters  IVariant=InternalParameters  DVariant=Disabled  IntegratorVariant=Continuous  SatVariant=Disabled  AWVariant=Passthrough  PCopyVariant=Disabled  TRVariant=Disabled  FdbkBlocksVariant=Forward  IdealPFdbkVariant=Disabled  SatFdbkVariant=Disabled  DerivativeFilterVariant=Disabled  NVariant=Disabled  NCopyVariant=Disabled_SignalSpec  FilterICVariant=Disabled  IntegratorICVariant=InternalICs  ExternalResetVariant=Disabled  TRSumVariant=Passthrough  SumFdbkVariant=Disabled  SumVariant=Sum_PI  TsampFilterVariant=InternalTs  TsampNgainVariant=Passthrough  TsampIntegralVariant=Passthrough
  Power (Positive-Sequence) : powerlib_meascontrol/Measurements/Power (Positive-Sequence)  Freq=50  Vinit=[1, 0]  Iinit=[1, 0]  Ts=1e-6
      settings: SourceProductBaseCode=PS
  Qcontr : Scope
  Saturation : Saturate  UpperLimit=20  LowerLimit=-20
  Saturation1 : Saturate  UpperLimit=20  LowerLimit=-20
  See1 : Scope
  To Workspace15 : ToWorkspace  VariableName=md1  SaveFormat=Timeseries  SampleTime=-1
  To Workspace16 : ToWorkspace  VariableName=mq1  SaveFormat=Timeseries  SampleTime=-1
  Vdc/1 : Constant  Value=400
  Vdc/2 : Constant  Value=400
  Vdc/3 : Constant  Value=0
  checksat1 : Scope
  checksat2 : Scope
  dq0 to abc : powerlib_meascontrol/Transformations/dq0 to abc  Alignment=90 degrees behind phase A axis
  ed : Scope
  eq : Scope
  err{1..4} (4 alike) : Scope
  m : Scope
  "md " : Scope
  mq : Scope
  reactive_droop_coef : Gain  Gain=0.05*230/13800
  ud : Scope
  uq : Scope
  mabc : Outport
  P : Outport  Port=2
  wires:
  Gain4/1 -> See1/1, Add1/3
  Add1/1 -> Divide2/1
  Vdc/2/1 -> Divide2/2
  Divide2/1 -> Mux/1, To Workspace15/1, "md "/1
  Add3/1 -> Divide3/1
  Vdc/1/1 -> Divide3/2
  Divide3/1 -> To Workspace16/1, mq/1, Mux/2
  Add4/1 -> eq/1, PID Controller1/1
  Vdc/3/1 -> Mux/3
  Add2/1 -> Saturation/1
  PID Controller1/1 -> uq/1, Add3/2
  PID Controller/1 -> ud/1, Add1/2
  Add/1 -> PID Controller/1, ed/1
  Add5/1 -> Saturation1/1
  Add6/1 -> err1/1, PID Controller2/1
  Vd/1 -> Gain3/1, Add1/1, Add6/1
  Constant1/1 -> Add7/2
  ILd/1 -> Gain1/1, Add/1, ILdscope/1
  Gain1/1 -> Add3/3
  Gain2/1 -> Add5/3
  Wt/1 -> dq0 to abc/2
  Gain3/1 -> Add2/2
  Mux/1 -> dq0 to abc/1
  ILq/1 -> Gain4/1, Add4/1
  dq0 to abc/1 -> mabc/1, m/1
  Iloadd/1 -> Add5/1
  Iloadq/1 -> Add2/3
  Saturation/1 -> checksat2/1, Add4/2
  Saturation1/1 -> checksat1/1, Add/2
  Vq/1 -> Add3/1, Add7/1, Gain2/1
  Add7/1 -> err2/1, PID Controller3/1
  PID Controller2/1 -> err4/1, Add5/2, err3/1
  PID Controller3/1 -> Add2/1
  Vsabc/1 -> Power (Positive-Sequence)/1
  Iloadabc/1 -> Power (Positive-Sequence)/2
  Power (Positive-Sequence)/2 -> reactive_droop_coef/1
  Power (Positive-Sequence)/1 -> P/1
  Constant/1 -> Add6/3
  reactive_droop_coef/1 -> Qcontr/1, Add6/2

== system BenchmarkModel_Dynamic_TestCase/VSI Converter1/Current Control ==
  note: current control
  P ref : Inport
  Q ref : Inport  Port=2
  Enable PI : Inport  Port=3
  Vabc_grid : Inport  Port=4
  Iabc_grid : Inport  Port=5
  Vabc_C : Inport  Port=6
  Iabc_C : Inport  Port=7
  SAT : Inport  Port=8
  Current Control : Subsystem
  Mux : Mux  Inputs=2
  Mux1 : Mux  Inputs=2
  PLL & Park Transformation : Subsystem
  Power (Positive-Sequence)2 : powerlib_meascontrol/Measurements/Power (Positive-Sequence)  Freq=50  Vinit=[0, 0]  Iinit=[0, 0]  Ts=0
      settings: SourceProductBaseCode=PS
  Pref --> Idref : Subsystem
  Qref --> Iqref : Subsystem
  Scope : Scope  NumInputPorts=2
  Scope1 : Scope  NumInputPorts=2
  Switch : Switch  Criteria=u2 > Threshold
  VSdq : Outport  VectorParamsAs1DForOutWhenUnconnected=off
  theta : Outport  Port=2
  wires:
  P ref/1 -> Scope/1, Pref --> Idref/1(P_rif)  "P ref"
  PLL & Park Transformation/9(f_grid) -> Qref --> Iqref/2(f_grid), Current Control/8(f_rete)
  SAT/1 -> Current Control/7(SAT)
  Current Control/1(VSd) -> Mux1/1
  Pref --> Idref/1(Id_rif) -> Current Control/5(Id_rif)  "Id ref"
  Qref --> Iqref/1(Iq_ref) -> Current Control/6(Iq_rif)
  Enable PI/1 -> Switch/2, Current Control/9(Enable PI)
  Mux1/1 -> Switch/1
  Mux/1 -> Switch/3
  Current Control/2(VSq) -> Mux1/2
  Switch/1 -> VSdq/1
  Power (Positive-Sequence)2/2 -> Scope1/2  "Q out"
  Power (Positive-Sequence)2/1 -> Scope/2  "P out"
  PLL & Park Transformation/1(Vabc) -> Power (Positive-Sequence)2/1
  PLL & Park Transformation/2(Iabc) -> Power (Positive-Sequence)2/2
  Q ref/1 -> Scope1/1, Qref --> Iqref/1(Q_ref)  "Q ref"
  Vabc_grid/1 -> PLL & Park Transformation/1(Vabc_grid)
  Iabc_grid/1 -> PLL & Park Transformation/2(Iabc_grid)
  Vabc_C/1 -> PLL & Park Transformation/3(Vabc_C)
  Iabc_C/1 -> PLL & Park Transformation/4(Iabc_C)
  PLL & Park Transformation/4(Vq) -> Mux/2, Current Control/4(Vcq), Pref --> Idref/3(Vq), Qref --> Iqref/5(Vq)
  PLL & Park Transformation/3(Vd) -> Pref --> Idref/4(Vd), Qref --> Iqref/3(Vd), Current Control/3(Vcd), Mux/1
  PLL & Park Transformation/6(Iq) -> Pref --> Idref/2(Iq), Current Control/2(Iq)
  PLL & Park Transformation/5(Id) -> Current Control/1(Id), Qref --> Iqref/4(Id)
  PLL & Park Transformation/7(VCd) -> Qref --> Iqref/6(VCd)
  PLL & Park Transformation/8(VCq) -> Qref --> Iqref/7(VCq)
  PLL & Park Transformation/10(theta) -> theta/1

== system BenchmarkModel_Dynamic_TestCase/VSI Converter1/Modulanti ==
  Vd : Inport
  Vq : Inport  Port=2
  Vdcbus : Inport  Port=3
  Theta : Inport  Port=4
  Complex to Magnitude-Angle : ComplexToMagnitudeAngle
  Complex to Real-Imag : ComplexToRealImag
  Constant : Constant  Value=0
  Divide : Product  Inputs=*/
  Magnitude-Angle to Complex : MagnitudeAngleToComplex
  Mux : Mux  Inputs=3
  Real-Imag to Complex : RealImagToComplex
  Saturation : Saturate  UpperLimit=1  LowerLimit=-1
  dq0 to abc : powerlib_meascontrol/Transformations/dq0 to abc  Alignment=90 degrees behind phase A axis
  mabc : Outport  VectorParamsAs1DForOutWhenUnconnected=off
  wires:
  Constant/1 -> Mux/3
  Mux/1 -> dq0 to abc/1
  dq0 to abc/1 -> Divide/1
  Vdcbus/1 -> Divide/2
  Divide/1 -> Saturation/1
  Real-Imag to Complex/1 -> Complex to Magnitude-Angle/1
  Vd/1 -> Real-Imag to Complex/1
  Vq/1 -> Real-Imag to Complex/2
  Complex to Magnitude-Angle/2 -> Magnitude-Angle to Complex/2
  Magnitude-Angle to Complex/1 -> Complex to Real-Imag/1
  Complex to Real-Imag/2 -> Mux/2
  Complex to Real-Imag/1 -> Mux/1
  Theta/1 -> dq0 to abc/2
  Saturation/1 -> mabc/1
  Complex to Magnitude-Angle/1 -> Magnitude-Angle to Complex/1

== system BenchmarkModel_Dynamic_TestCase/Subsystem/Three-Phase Tap Changer Transformer Pn MVA, Up // Us kV/Tap Changer Control ==
  "Up " : Inport
  "Down " : Inport  Port=2
  Constant : Constant  Value=-1
  Constant1 : Constant
  Determine tap position : Subsystem
  Edge Detector : Subsystem  DialogController=POWERSYS.PowerSysDialog  mask(Edge Detector){model=Rising, ic=0}
      mask prompts: model "Edge:"; ic "Input at t = -eps:"
      mask help:
      | This block compares its present input to its previous input.
      |
      | If the input  is a logic signal (TRUE (1) or FALSE (0), the output is a one-step boolean signal TRUE  when  the specified edge (Rising, Falling or Either)  is detected.
      |
      | This block can also be used to detect the slope polarity of a continuous signal. For example, if the specified edge is  "Rising", the output is TRUE as long as the slope of the input signal is positive.
      |
      | The input value at time preceding t=0 is specified by the parameter "Input at t=-eps"
      mask init:
      | if model~=3,
      | 	x1 = (model -1)*20;
      |     x2 = (model -1)*60;
      | 	X1=[5,20,20,35]+25; Y1=[20+x2,20+x2,80-x2,80-x2];
      | 	X2=[5,20,35]+25;    Y2=[40+x1,60-x1,40+x1];
      | 	X3=[];X4=[];Y3=[];Y4=[];
      | else
      | 	x1 = 20;
      | 	x2 = 60;
      | 	X1=[5,20,20,35]+8; Y1=[20,20,80,80];
      | 	X2=[5,20,35]+8;    Y2=[40,60,40];
      | 	X3=[5,20,20,35]+53; Y3=[20+x2,20+x2,80-x2,80-x2];
      | 	X4=[5,20,35]+53;    Y4=[40+x1,60-x1,40+x1];
      | end
      | power_initmask();
      mask Help: This block is part of a subset of blocks in the Extras library that does not have documentation associated with it, other than the block mask description.
      mask TypeOptions model: Rising | Falling | Either
      mask Display: plot(0,0,100,100, X1,Y1,X2,Y2,X3,Y3,X4,Y4);
  Logical Operator : Logic  Operator=OR  AllPortsSameDT=off
  Logical Operator1 : Logic  AllPortsSameDT=off
  Mechanical Delay : TransportDelay  DelayTime=MecDelay  InitialOutput=InitialPosition  BufferSize=5120
  Memory : Memory  InitialCondition=1  InheritSampleTime=on
  Relational Operator : RelationalOperator  Operator===  OutDataTypeStr=float('double')  RndMeth=Nearest
  Switch : Switch  Threshold=0.5  SaturateOnIntegerOverflow=on
  TapNo : Outport  VectorParamsAs1DForOutWhenUnconnected=off
  Ready : Outport  Port=2  VectorParamsAs1DForOutWhenUnconnected=off
  wires:
  Edge Detector/1(Out) -> Logical Operator1/2
  Logical Operator/1 -> Edge Detector/1(In)
  Memory/1 -> Ready/1, Logical Operator1/1
  Relational Operator/1 -> Memory/1
  Determine tap position/1(TapNo) -> Relational Operator/1, Mechanical Delay/1
  Switch/1 -> Determine tap position/1(NewTap)
  Constant1/1 -> Switch/3
  Constant/1 -> Switch/1
  "Down "/1 -> Switch/2, Logical Operator/2
  "Up "/1 -> Logical Operator/1
  Logical Operator1/1 -> Determine tap position/Trigger
  Mechanical Delay/1 -> Relational Operator/2, TapNo/1

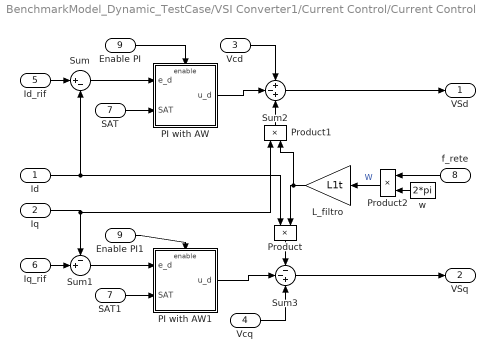
== system BenchmarkModel_Dynamic_TestCase/VSI Converter1/Current Control/Current Control ==
  Id : Inport
  Iq : Inport  Port=2
  Vcd : Inport  Port=3
  Vcq : Inport  Port=4
  Id_rif : Inport  Port=5
  Iq_rif : Inport  Port=6
  SAT : Inport  Port=7
  f_rete : Inport  Port=8
  Enable PI : Inport  Port=9
  Enable PI1 : InportShadow  Port=9
  L_filtro : Gain  Gain=L1t
  PI with AW : Subsystem  mask{PI_KP=9.4, PI_KI=146}
      mask prompts: PI_KP "Kp"; PI_KI "Ki"
      mask Display: disp(' ');
  PI with AW1 : Subsystem  mask{PI_KP=9.4, PI_KI=146}
      mask prompts: PI_KP "Kp"; PI_KI "Ki"
      mask Display: disp(' ');
  Product : Product
  Product1 : Product
  Product2 : Product
  SAT1 : InportShadow  Port=7
  Sum : Sum  Inputs=|+-
  Sum1 : Sum  Inputs=-+|
  Sum2 : Sum  Inputs=+-+
  Sum3 : Sum  Inputs=--+
  w : Constant  Value=2*pi
  VSd : Outport  VectorParamsAs1DForOutWhenUnconnected=off
  VSq : Outport  Port=2  VectorParamsAs1DForOutWhenUnconnected=off
  wires:
  Id_rif/1 -> Sum/1
  Id/1 -> Sum/2, Product/1
  Sum/1 -> PI with AW/1(e_d)
  Sum1/1 -> PI with AW1/1(e_d)
  PI with AW/1(u_d) -> Sum2/2
  PI with AW1/1(u_d) -> Sum3/2
  Iq_rif/1 -> Sum1/2
  Iq/1 -> Sum1/1, Product1/1
  L_filtro/1 -> Product1/2, Product/2
  Vcq/1 -> Sum3/3
  Vcd/1 -> Sum2/1
  Sum2/1 -> VSd/1
  Sum3/1 -> VSq/1
  Product/1 -> Sum3/1
  Product1/1 -> Sum2/3
  Product2/1 -> L_filtro/1  "W"
  w/1 -> Product2/2
  f_rete/1 -> Product2/1
  SAT/1 -> PI with AW/2(SAT)
  SAT1/1 -> PI with AW1/2(SAT)
  Enable PI/1 -> PI with AW/Enable
  Enable PI1/1 -> PI with AW1/Enable

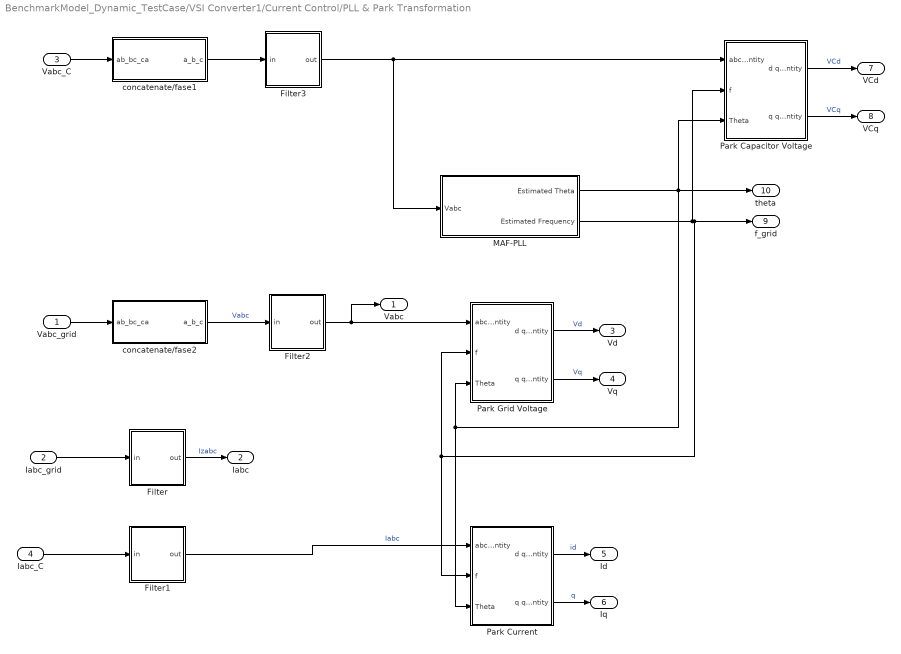
== system BenchmarkModel_Dynamic_TestCase/VSI Converter1/Current Control/PLL & Park Transformation ==
  Vabc_grid : Inport
  Iabc_grid : Inport  Port=2
  Vabc_C : Inport  Port=3
  Iabc_C : Inport  Port=4
  Filter : Subsystem  mask{Ft=500}
      mask prompts: Ft "Filter Frequency [Hz]"
  Filter1 : Subsystem  mask{Ft=500}
      mask prompts: Ft "Filter Frequency [Hz]"
  Filter2 : Subsystem  mask{Ft=500}
      mask prompts: Ft "Filter Frequency [Hz]"
  Filter3 : Subsystem  mask{Ft=500}
      mask prompts: Ft "Filter Frequency [Hz]"
  MAF-PLL : Subsystem  mask{Kp_PLL=80, Ki_PLL=1000, Tw=0.01, initPhase=0, initFreq=50, Non_limited_theta=on}
      mask prompts: Kp_PLL "Kp"; Ki_PLL "Ki"; initPhase "Set initial estimated phase (degrees)"; initFreq "Set initial estimated frequency (Hz)"; Non_limited_theta "Check if desired unlimited theta, otherwise it will be limited between 0 and 2*pi"
      mask DialogControl QT1_PLL Prompt: QuasiType1 PLL
      mask DialogControl QT1_PLL_descr Prompt: Kp is proportional gain of the PLL while Tw the window width of the MAF used to filter out d and q
  Park Capacitor Voltage : Subsystem  mask{Ft=500}
      mask prompts: Ft "Filter Frequency [Hz]"
  Park Current : Subsystem  mask{Ft=500}
      mask prompts: Ft "Filter Frequency [Hz]"
  Park Grid Voltage : Subsystem  mask{Ft=500}
      mask prompts: Ft "Filter Frequency [Hz]"
  concatenate/fase1 : Subsystem
  concatenate/fase2 : Subsystem
  Vabc : Outport  VectorParamsAs1DForOutWhenUnconnected=off
  Iabc : Outport  Port=2  VectorParamsAs1DForOutWhenUnconnected=off
  Vd : Outport  Port=3
  Vq : Outport  Port=4
  Id : Outport  Port=5
  Iq : Outport  Port=6
  VCd : Outport  Port=7
  VCq : Outport  Port=8
  f_grid : Outport  Port=9
  theta : Outport  Port=10
  wires:
  Filter3/1(out) -> Park Capacitor Voltage/1(abc quantity), MAF-PLL/1(Vabc)
  Filter2/1(out) -> Park Grid Voltage/1(abc quantity), Vabc/1
  Iabc_C/1 -> Filter1/1(in)
  Filter1/1(out) -> Park Current/1(abc quantity)  "Iabc"
  Vabc_C/1 -> concatenate/fase1/1(ab_bc_ca)
  concatenate/fase2/1(a_b_c) -> Filter2/1(in)  "Vabc"
  Vabc_grid/1 -> concatenate/fase2/1(ab_bc_ca)
  Iabc_grid/1 -> Filter/1(in)
  Filter/1(out) -> Iabc/1  "Izabc"
  Park Grid Voltage/1(d quantity) -> Vd/1  "Vd"
  Park Grid Voltage/2(q quantity) -> Vq/1  "Vq"
  Park Current/2(q quantity) -> Iq/1  "q"
  Park Current/1(d quantity) -> Id/1  "id"
  Park Capacitor Voltage/1(d quantity) -> VCd/1  "VCd"
  Park Capacitor Voltage/2(q quantity) -> VCq/1  "VCq"
  concatenate/fase1/1(a_b_c) -> Filter3/1(in)
  MAF-PLL/1(Estimated Theta) -> theta/1, Park Current/3(Theta), Park Grid Voltage/3(Theta), Park Capacitor Voltage/3(Theta)
  MAF-PLL/2(Estimated Frequency) -> f_grid/1, Park Current/2(f), Park Grid Voltage/2(f), Park Capacitor Voltage/2(f)

== system BenchmarkModel_Dynamic_TestCase/VSI Converter1/Current Control/Pref --> Idref ==
  P_rif : Inport
  Iq : Inport  Port=2
  Vq : Inport  Port=3
  Vd : Inport  Port=4
  Add : Sum  Inputs=+-
  Divide : Product  Inputs=*/
  Gain : Gain  Gain=2/3
  Product : Product
  Saturation1 : Saturate  UpperLimit=Pmax  LowerLimit=-Pmax
  Id_rif : Outport  VectorParamsAs1DForOutWhenUnconnected=off
  wires:
  P_rif/1 -> Saturation1/1
  Gain/1 -> Add/1
  Iq/1 -> Product/1
  Vq/1 -> Product/2
  Product/1 -> Add/2
  Add/1 -> Divide/1
  Vd/1 -> Divide/2
  Divide/1 -> Id_rif/1
  Saturation1/1 -> Gain/1

== system BenchmarkModel_Dynamic_TestCase/VSI Converter1/Current Control/Qref --> Iqref ==
  Q_ref : Inport
  f_grid : Inport  Port=2
  Vd : Inport  Port=3
  Id : Inport  Port=4
  Vq : Inport  Port=5
  VCd : Inport  Port=6
  VCq : Inport  Port=7
  Add : Sum  Inputs=-+
  Add1 : Sum
  Divide : Product  Inputs=*/
  Filter Compensation : MATLAB Function  TreatAsAtomicUnit=on
  Gain : Gain  Gain=2/3
  Parameter : Subsystem
  Product : Product
  Saturation2 : Saturate  UpperLimit=Qmax  LowerLimit=-Qmax
  Transfer Fcn1 : TransferFcn  Denominator=[1/300 1]
  Vc : Subsystem
  Iq_ref : Outport  VectorParamsAs1DForOutWhenUnconnected=off
  wires:
  Divide/1 -> Iq_ref/1
  Vd/1 -> Divide/2
  Add/1 -> Divide/1
  Product/1 -> Add/2
  Gain/1 -> Add/1
  Vq/1 -> Product/1
  Id/1 -> Product/2
  Vc/1(Vc_rms) -> Filter Compensation/2(Vc)
  Transfer Fcn1/1 -> Add1/2
  Add1/1 -> Saturation2/1
  Parameter/1(Parameters) -> Filter Compensation/3(Param)
  Filter Compensation/1(Qc) -> Transfer Fcn1/1
  f_grid/1 -> Filter Compensation/1(f)
  Q_ref/1 -> Add1/1  "Q ref"
  Saturation2/1 -> Gain/1
  VCd/1 -> Vc/1(VCd)
  VCq/1 -> Vc/2(VCq)

== system BenchmarkModel_Dynamic_TestCase/Subsystem/Three-Phase Tap Changer Transformer Pn MVA, Up // Us kV/Tap Changer Control/Determine tap position ==
  NewTap : Inport
  Trigger : TriggerPort  VariantControl=Variant
  Memory : Memory  InitialCondition=InitialPosition  InheritSampleTime=on
  Saturation : Saturate  UpperLimit=MinMaxTap(2)  LowerLimit=MinMaxTap(1)
  Sum : Sum  Inputs=|++  SaturateOnIntegerOverflow=on
  TapNo : Outport  InitialOutput=InitialPosition  VectorParamsAs1DForOutWhenUnconnected=off
  wires:
  Saturation/1 -> Memory/1, TapNo/1
  Memory/1 -> Sum/2
  Sum/1 -> Saturation/1
  NewTap/1 -> Sum/1

== system BenchmarkModel_Dynamic_TestCase/Subsystem/Three-Phase Tap Changer Transformer Pn MVA, Up // Us kV/Tap Changer Control/Edge Detector ==
  note: Edge or Slope Detector
  In : Inport
  Constant1 : Constant  Value=model
  Demux : Demux  Outputs=2
      settings: DisplayOption=none
  Logical Operator1 : Logic  Operator=OR
  Memory : Memory  InitialCondition=ic  LinearizeAsDelay=on
  Multiport Switch : MultiPortSwitch  SaturateOnIntegerOverflow=on
  NEGATIVE Edge : Subsystem  TreatAsAtomicUnit=on
  POSITIVE Edge : Subsystem  TreatAsAtomicUnit=on
  either edge : Constant  Value=[1 1]
  neg. edge : Constant  Value=[0 1]
  pos. edge : Constant  Value=[1 0]
  Out : Outport  VectorParamsAs1DForOutWhenUnconnected=off
  wires:
  Logical Operator1/1 -> Out/1
  NEGATIVE Edge/1(OUT) -> Logical Operator1/2
  POSITIVE Edge/1(OUT) -> Logical Operator1/1
  Memory/1 -> POSITIVE Edge/2(IN previous), NEGATIVE Edge/2(IN previous)
  In/1 -> POSITIVE Edge/1(IN), NEGATIVE Edge/1(IN), Memory/1
  pos. edge/1 -> Multiport Switch/2
  neg. edge/1 -> Multiport Switch/3
  Constant1/1 -> Multiport Switch/1
  Multiport Switch/1 -> Demux/1
  Demux/1 -> POSITIVE Edge/Enable
  Demux/2 -> NEGATIVE Edge/Enable
  either edge/1 -> Multiport Switch/4

== system BenchmarkModel_Dynamic_TestCase/VSI Converter1/Current Control/Current Control/PI with AW ==
  e_d : Inport
  SAT : Inport  Port=2
  Enable : EnablePort
  Constant : Constant  Value=0
  Integrator : Integrator
  Ki : Gain  Gain=PI_KI
  Kp : Gain  Gain=PI_KP
  Logical Operator : Logic  Operator=NOT  AllPortsSameDT=off  OutDataTypeStr=boolean
  Sum : Sum  Inputs=|++
  Switch : Switch  Criteria=u2 > Threshold
  u_d : Outport  VectorParamsAs1DForOutWhenUnconnected=off
  wires:
  e_d/1 -> Switch/1, Kp/1
  Sum/1 -> u_d/1
  Kp/1 -> Sum/1
  Integrator/1 -> Ki/1
  Switch/1 -> Integrator/1
  Constant/1 -> Switch/3
  SAT/1 -> Logical Operator/1
  Ki/1 -> Sum/2
  Logical Operator/1 -> Switch/2

== system BenchmarkModel_Dynamic_TestCase/VSI Converter1/Current Control/Current Control/PI with AW1 ==
  e_d : Inport
  SAT : Inport  Port=2
  Enable : EnablePort
  Constant : Constant  Value=0
  Integrator : Integrator
  Ki : Gain  Gain=PI_KI
  Kp : Gain  Gain=PI_KP
  Logical Operator : Logic  Operator=NOT  AllPortsSameDT=off  OutDataTypeStr=boolean
  Sum : Sum  Inputs=|++
  Switch : Switch  Criteria=u2 > Threshold
  u_d : Outport  VectorParamsAs1DForOutWhenUnconnected=off
  wires:
  e_d/1 -> Switch/1, Kp/1
  Sum/1 -> u_d/1
  Kp/1 -> Sum/1
  Integrator/1 -> Ki/1
  Switch/1 -> Integrator/1
  Constant/1 -> Switch/3
  SAT/1 -> Logical Operator/1
  Ki/1 -> Sum/2
  Logical Operator/1 -> Switch/2

== system BenchmarkModel_Dynamic_TestCase/VSI Converter1/Current Control/PLL & Park Transformation/Filter ==
  in : Inport
  Demux : Demux  Outputs=3
  Mux : Mux  Inputs=3
  Transfer Fcn1 : TransferFcn  Denominator=[1/(2*pi*Ft) 1]
  Transfer Fcn2 : TransferFcn  Denominator=[1/(2*pi*Ft) 1]
  Transfer Fcn3 : TransferFcn  Denominator=[1/(2*pi*Ft) 1]
  out : Outport  VectorParamsAs1DForOutWhenUnconnected=off
  wires:
  Mux/1 -> out/1
  in/1 -> Demux/1
  Transfer Fcn3/1 -> Mux/3
  Transfer Fcn2/1 -> Mux/2
  Transfer Fcn1/1 -> Mux/1
  Demux/3 -> Transfer Fcn3/1
  Demux/1 -> Transfer Fcn1/1
  Demux/2 -> Transfer Fcn2/1

== system BenchmarkModel_Dynamic_TestCase/VSI Converter1/Current Control/PLL & Park Transformation/Filter1 ==
  in : Inport
  Demux : Demux  Outputs=3
  Mux : Mux  Inputs=3
  Transfer Fcn1 : TransferFcn  Denominator=[1/(2*pi*Ft) 1]
  Transfer Fcn2 : TransferFcn  Denominator=[1/(2*pi*Ft) 1]
  Transfer Fcn3 : TransferFcn  Denominator=[1/(2*pi*Ft) 1]
  out : Outport  VectorParamsAs1DForOutWhenUnconnected=off
  wires:
  Demux/2 -> Transfer Fcn2/1
  Demux/1 -> Transfer Fcn1/1
  Demux/3 -> Transfer Fcn3/1
  Transfer Fcn1/1 -> Mux/1
  Transfer Fcn2/1 -> Mux/2
  Transfer Fcn3/1 -> Mux/3
  in/1 -> Demux/1
  Mux/1 -> out/1
